simulink model "roll_loop"  (R2016a)
settings: Solver=VariableStepAuto  StartTime=0.0  StopTime=10.0  RelTol=1e-3
undefined symbols (not defined in the file or in its folder): a_phi1, a_phi2, roll_kd, roll_kp
settings Model: Creator=andreanv  LastModifiedBy=andreanv

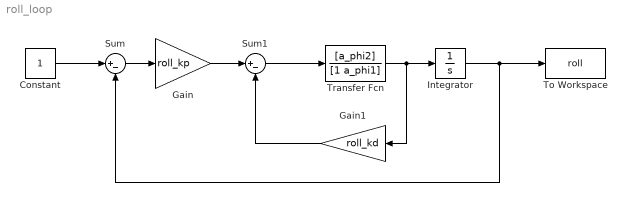
== system roll_loop ==
  Constant : Constant
  Gain : Gain  Gain=roll_kp
  Gain1 : Gain  Gain=roll_kd
  Integrator : Integrator
  Sum : Sum  Inputs=|+-
  Sum1 : Sum  Inputs=|+-
  To Workspace : ToWorkspace  VariableName=roll  SaveFormat=Timeseries  SampleTime=-1
  Transfer Fcn : TransferFcn  Numerator=[a_phi2]  Denominator=[1 a_phi1]
  wires:
  Constant/1 -> Sum/1
  Sum/1 -> Gain/1
  Gain/1 -> Sum1/1
  Sum1/1 -> Transfer Fcn/1
  Gain1/1 -> Sum1/2
  Transfer Fcn/1 -> Gain1/1, Integrator/1
  Integrator/1 -> Sum/2, To Workspace/1
